simulink model "ObstacleControl"  (R2020a)
settings: Solver=ode3  StartTime=0.0  StopTime=10.0  RelTol=1e-3
PreLoadFcn:
  | % Lidar parameters
  | 
  | 
  | scanAngles = linspace(-pi/2,pi/2,360);
  | scanMaxRange = 3.5;
  | scanSensorOffset = [0,0];
model workspace (MAT data in the model file):
  destX = 2
  destY = 2
undefined symbols (not defined in the file or in its folder): Angular, Linear
libraries: robotlib x8, simulink x2, robotalgslib x2, robotcorelib x1
settings Model: Creator=Pierre  LastModifiedBy=pierre
settings OptimizationCC: EnhancedBackFolding=on  PassReuseOutputArgsAs=Individual arguments  ZeroExternalMemoryAtStartup=off  ZeroInternalMemoryAtStartup=off  MaxStackSize=64  OptimizeBlockOrder=speed  DifferentSizesBufferReuse=on  OptimizationCustomize=off  EfficientTunableParamExpr=on
settings DebuggingCC: ParameterTunabilityLossMsg=error
settings HardwareCC: ProdBitPerPointer=32  ProdBitPerSizeT=32  ProdBitPerPtrDiffT=32  ProdLargestAtomicFloat=None  ProdIntDivRoundTo=Undefined  ProdEndianess=Unspecified  ProdWordSize=32  ProdHWDeviceType=Generic->Unspecified (assume 32-bit Generic)
settings SFSimCC: MATLABDynamicMemAlloc=off
settings RTWCC: SystemTargetFile=ert.tlc  HardwareBoard=Robot Operating System (ROS)  TemplateMakefile=ert_default_tmf  Toolchain=Catkin  TargetLang=C++
settings CodeAppCC: ForceParamTrailComments=on  IgnoreCustomStorageClasses=off  OperatorAnnotations=on  SimulinkDataObjDesc=on  SFDataObjDesc=on  InsertBlockDesc=on
settings ERTTargetCC: SupportVariableSizeSignals=on

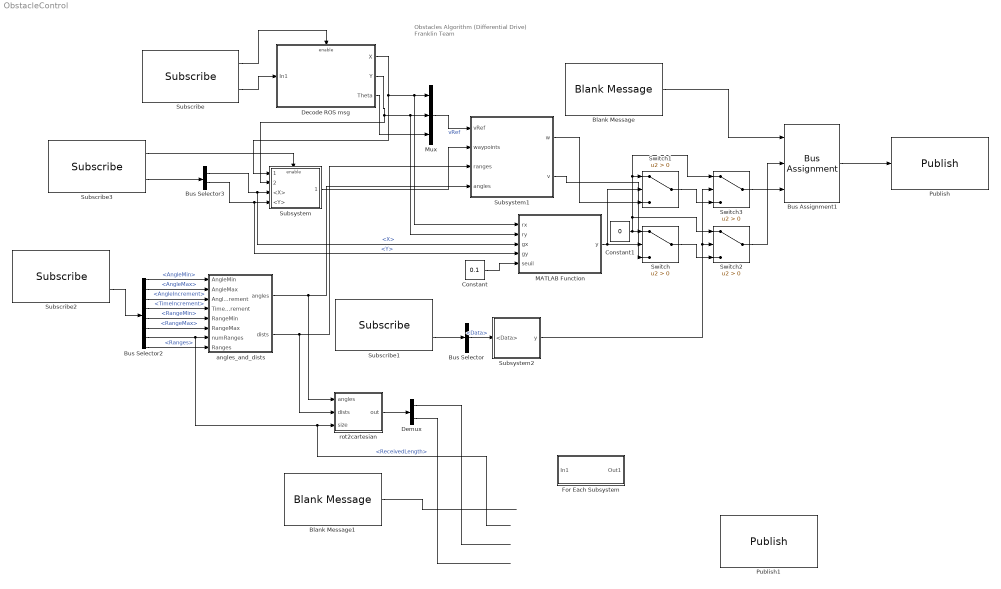
== system ObstacleControl ==
  note: Obstacles Algorithm
      | (Differential Drive)
      |
      | Franklin Team
  Blank Message : robotlib/Blank Message  messageClass=Message  entityType=geometry_msgs/Twist  messageType=geometry_msgs/Twist  SampleTime=inf
  Blank Message1 : robotlib/Blank Message  messageClass=Message  entityType=sensor_msgs/PointCloud  messageType=sensor_msgs/PointCloud  SampleTime=inf
  Bus Assignment1 : BusAssignment  AssignedSignals=Linear.X,Angular.Z
  Bus Selector : BusSelector  DialogController=Simulink.DDGSource_BusSelector  OutputSignals=Data
  Bus Selector2 : BusSelector  OutputSignals=AngleMin,AngleMax,AngleIncrement,TimeIncrement,RangeMin,RangeMax,Ranges_SL_Info.ReceivedLength,Ranges
  Bus Selector3 : BusSelector  OutputSignals=X,Y
  Constant : Constant  Value=0.1
  Constant1 : Constant  Value=0
  Decode ROS msg : Subsystem
  Demux : Demux  Outputs=2
  For Each Subsystem : Subsystem  TreatAsAtomicUnit=on
  MATLAB Function : MATLAB Function  TreatAsAtomicUnit=on
  Mux : Mux  Inputs=3
  Publish : robotlib/Publish  topicSource=Specify your own  topic=/cmd_vel  messageType=geometry_msgs/Twist  messageQueueLength=1
  Publish1 : robotlib/Publish  topicSource=Specify your own  topic=/modelScan  messageType=sensor_msgs/PointCloud  messageQueueLength=1
  Subscribe : robotlib/Subscribe  topicSource=Specify your own  topic=/odom  messageType=nav_msgs/Odometry  sampleTime=-1  messageQueueLength=1
  Subscribe1 : robotlib/Subscribe  topicSource=Specify your own  topic=/destination/stop  messageType=std_msgs/Bool  sampleTime=1  messageQueueLength=1
  Subscribe2 : robotlib/Subscribe  topicSource=Specify your own  topic=/scan  messageType=sensor_msgs/LaserScan  sampleTime=1  messageQueueLength=1
  Subscribe3 : robotlib/Subscribe  topicSource=Specify your own  topic=/destination  messageType=geometry_msgs/Pose2D  sampleTime=1  messageQueueLength=1
  Subsystem : Subsystem
  Subsystem1 : Subsystem
  Subsystem2 : Subsystem
  Switch{,1..3} (4 alike) : Switch  Criteria=u2 > Threshold
  angles_and_dists : MATLAB Function  TreatAsAtomicUnit=on
  rot2cartesian : MATLAB Function  TreatAsAtomicUnit=on
  wires:
  Blank Message/1 -> Bus Assignment1/1
  Bus Assignment1/1 -> Publish/1
  Subscribe3/2 -> Bus Selector3/1
  Subscribe3/1 -> Subsystem/Enable
  Subscribe/2 -> Decode ROS msg/1(In1)
  Subscribe/1 -> Decode ROS msg/Enable
  Decode ROS msg/1(X) -> Subsystem/1(<Xinit>), MATLAB Function/1(rx), Mux/1
  Decode ROS msg/2(Y) -> Subsystem/2(<Yinit>), MATLAB Function/2(ry), Mux/2
  Decode ROS msg/3(Theta) -> Mux/3
  Bus Selector3/1 -> MATLAB Function/3(gx), Subsystem/3(<X>)  "<X>"
  Bus Selector3/2 -> MATLAB Function/4(gy), Subsystem/4(<Y>)  "<Y>"
  Constant/1 -> MATLAB Function/5(seuil)
  MATLAB Function/1(y) -> Switch1/2, Switch/2
  Constant1/1 -> Switch2/1, Switch3/1, Switch1/1, Switch/1
  Switch/1 -> Switch2/3
  Switch2/1 -> Bus Assignment1/2
  Switch1/1 -> Switch3/3
  Switch3/1 -> Bus Assignment1/3
  Subscribe1/2 -> Bus Selector/1
  Subsystem2/1(y) -> Switch2/2, Switch3/2
  Bus Selector/1 -> Subsystem2/1(<Data>)  "<Data>"
  Subscribe2/2 -> Bus Selector2/1
  Mux/1 -> Subsystem1/1(vRef)  "vRef"
  Subsystem/1(waypoints) -> Subsystem1/2(waypoints)
  Subsystem1/1(w) -> Switch1/3
  Subsystem1/2(v) -> Switch/3
  Bus Selector2/6 -> angles_and_dists/6(RangeMax)  "<RangeMax>"
  Bus Selector2/2 -> angles_and_dists/2(AngleMax)  "<AngleMax>"
  Bus Selector2/3 -> angles_and_dists/3(AngleIncrement)  "<AngleIncrement>"
  Bus Selector2/5 -> angles_and_dists/5(RangeMin)  "<RangeMin>"
  Bus Selector2/7 -> rot2cartesian/3(size), angles_and_dists/7(numRanges)  "<ReceivedLength>"
  Bus Selector2/8 -> angles_and_dists/8(Ranges)  "<Ranges>"
  Bus Selector2/1 -> angles_and_dists/1(AngleMin)  "<AngleMin>"
  Bus Selector2/4 -> angles_and_dists/4(TimeIncrement)  "<TimeIncrement>"
  angles_and_dists/2(dists) -> rot2cartesian/2(dists), Subsystem1/3(ranges)
  angles_and_dists/1(angles) -> rot2cartesian/1(angles), Subsystem1/4(angles)
  Blank Message1/1 -> ?
  rot2cartesian/1(out) -> Demux/1
  Demux/1 -> ?
  Demux/2 -> ?
  ? -> Publish1/1

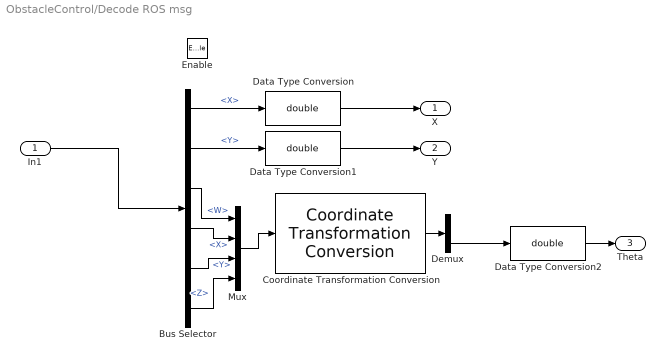
== system ObstacleControl/Decode ROS msg ==
  In1 : Inport
  Enable : EnablePort
  Bus Selector : BusSelector  DialogController=Simulink.DDGSource_BusSelector  OutputSignals=Pose.Pose.Position.X,Pose.Pose.Position.Y,Pose.Pose.Orientation.W,Pose.Pose.Orientation.X,Pose.Pose.Orientation.Y,Pose.Pose.Orientation.Z
  Coordinate Transformation Conversion : robotcorelib/Coordinate Transformation Conversion  InputRepresentation=Quaternion  InputEulerSequence=ZYX  ShowTrVecInputPort=on  OutputRepresentation=Euler Angles  OutputEulerSequence=XYZ  ShowTrVecOutputPort=on  SimulateUsing=Interpreted execution
      settings: SourceProductBaseCode=NV,RO,RR
  Data Type Conversion : DataTypeConversion  OutDataTypeStr=double
  Data Type Conversion1 : DataTypeConversion  OutDataTypeStr=double
  Data Type Conversion2 : DataTypeConversion  OutDataTypeStr=double
  Demux : Demux  Outputs=3
  Mux : Mux
  X : Outport  VectorParamsAs1DForOutWhenUnconnected=off
  Y : Outport  Port=2  VectorParamsAs1DForOutWhenUnconnected=off
  Theta : Outport  Port=3  VectorParamsAs1DForOutWhenUnconnected=off
  wires:
  In1/1 -> Bus Selector/1
  Bus Selector/2 -> Data Type Conversion1/1  "<Y>"
  Bus Selector/1 -> Data Type Conversion/1  "<X>"
  Data Type Conversion/1 -> X/1
  Data Type Conversion1/1 -> Y/1
  Data Type Conversion2/1 -> Theta/1
  Bus Selector/3 -> Mux/1  "<W>"
  Bus Selector/4 -> Mux/2  "<X>"
  Bus Selector/5 -> Mux/3  "<Y>"
  Bus Selector/6 -> Mux/4  "<Z>"
  Mux/1 -> Coordinate Transformation Conversion/1
  Coordinate Transformation Conversion/1 -> Demux/1
  Demux/3 -> Data Type Conversion2/1

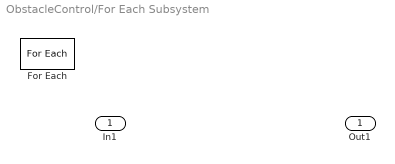
== system ObstacleControl/For Each Subsystem ==
  In1 : Inport  Partition=on  PartitionDimension=1  PartitionWidth=1  PartitionOffset=0
  For Each : ForEach  DisableCoverage=on
  Out1 : Outport  ConcatenationDimension=1

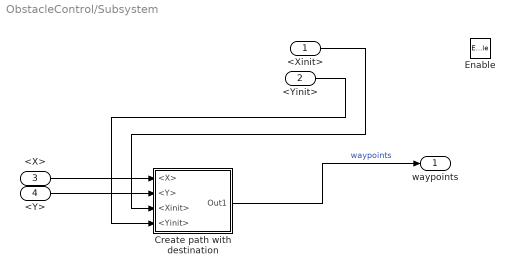
== system ObstacleControl/Subsystem ==
  <Xinit> : Inport
  <Yinit> : Inport  Port=2
  <X> : Inport  Port=3
  <Y> : Inport  Port=4
  Enable : EnablePort
  Create path with destination : Subsystem
  waypoints : Outport
  wires:
  <Yinit>/1 -> Create path with destination/4(<Yinit>)
  <X>/1 -> Create path with destination/1(<X>)
  <Y>/1 -> Create path with destination/2(<Y>)
  Create path with destination/1(Out1) -> waypoints/1  "waypoints"
  <Xinit>/1 -> Create path with destination/3(<Xinit>)

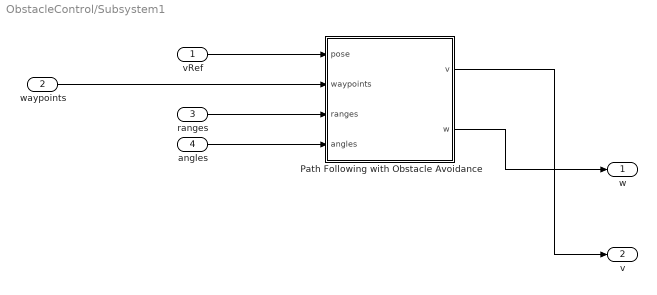
== system ObstacleControl/Subsystem1 ==
  vRef : Inport
  waypoints : Inport  Port=2
  ranges : Inport  Port=3
  angles : Inport  Port=4
  Path Following with Obstacle Avoidance : Subsystem
  w : Outport
  v : Outport  Port=2
  wires:
  vRef/1 -> Path Following with Obstacle Avoidance/1(pose)
  Path Following with Obstacle Avoidance/2(w) -> w/1
  waypoints/1 -> Path Following with Obstacle Avoidance/2(waypoints)
  Path Following with Obstacle Avoidance/1(v) -> v/1
  ranges/1 -> Path Following with Obstacle Avoidance/3(ranges)
  angles/1 -> Path Following with Obstacle Avoidance/4(angles)

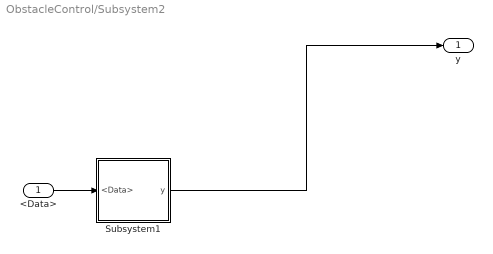
== system ObstacleControl/Subsystem2 ==
  <Data> : Inport
  Subsystem1 : Subsystem
  y : Outport
  wires:
  Subsystem1/1(y) -> y/1
  <Data>/1 -> Subsystem1/1(<Data>)

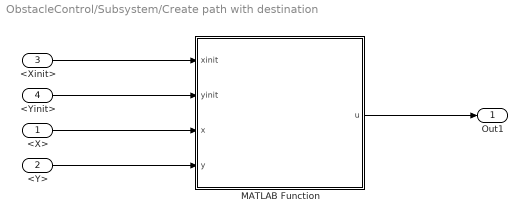
== system ObstacleControl/Subsystem/Create path with destination ==
  <X> : Inport
  <Y> : Inport  Port=2
  <Xinit> : Inport  Port=3
  <Yinit> : Inport  Port=4
  MATLAB Function : MATLAB Function  TreatAsAtomicUnit=on
  Out1 : Outport
  wires:
  <Y>/1 -> MATLAB Function/4(y)
  <X>/1 -> MATLAB Function/3(x)
  MATLAB Function/1(u) -> Out1/1
  <Xinit>/1 -> MATLAB Function/1(xinit)
  <Yinit>/1 -> MATLAB Function/2(yinit)

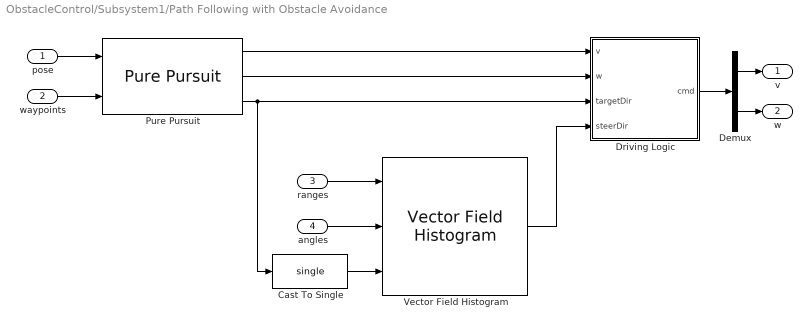
== system ObstacleControl/Subsystem1/Path Following with Obstacle Avoidance ==
  pose : Inport
  waypoints : Inport  Port=2
  ranges : Inport  Port=3
  angles : Inport  Port=4
  Cast To Single : DataTypeConversion  OutDataTypeStr=single
  Demux : Demux  Outputs=2
  Driving Logic : Subsystem
  Pure Pursuit : robotalgslib/Pure Pursuit  DesiredLinearVelocity=0.1  MaxAngularVelocity=1.5  LookaheadDistance=0.2  TargetDirPort=on  SimulateUsing=Interpreted execution
      settings: SourceProductBaseCode=RO
  Vector Field Histogram : robotalgslib/Vector Field Histogram  NumAngularSectors=36  DistanceLimits=[ 0.05, 3 ]  HistogramThresholds=[ 5, 10 ]  RobotRadius=0.1  SafetyDistance=0.2  MinTurningRadius=0.25  SimulateUsing=Interpreted execution  TargetDirectionWeight=5  CurrentDirectionWeight=2  PreviousDirectionWeight=2
      settings: SourceProductBaseCode=RO
  v : Outport  VectorParamsAs1DForOutWhenUnconnected=off
  w : Outport  Port=2  VectorParamsAs1DForOutWhenUnconnected=off
  wires:
  pose/1 -> Pure Pursuit/1
  Pure Pursuit/3 -> Driving Logic/3(targetDir), Cast To Single/1
  Pure Pursuit/1 -> Driving Logic/1(v)
  angles/1 -> Vector Field Histogram/2
  Vector Field Histogram/1 -> Driving Logic/4(steerDir)
  ranges/1 -> Vector Field Histogram/1
  waypoints/1 -> Pure Pursuit/2
  Pure Pursuit/2 -> Driving Logic/2(w)
  Demux/1 -> v/1
  Demux/2 -> w/1
  Driving Logic/1(cmd) -> Demux/1
  Cast To Single/1 -> Vector Field Histogram/3

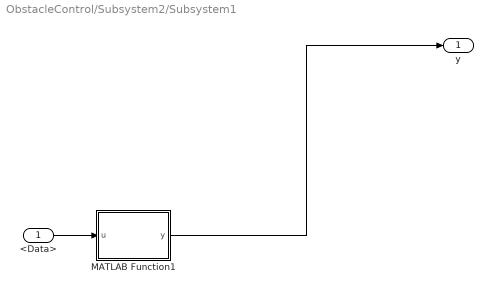
== system ObstacleControl/Subsystem2/Subsystem1 ==
  <Data> : Inport
  MATLAB Function1 : MATLAB Function  TreatAsAtomicUnit=on
  y : Outport
  wires:
  <Data>/1 -> MATLAB Function1/1(u)
  MATLAB Function1/1(y) -> y/1

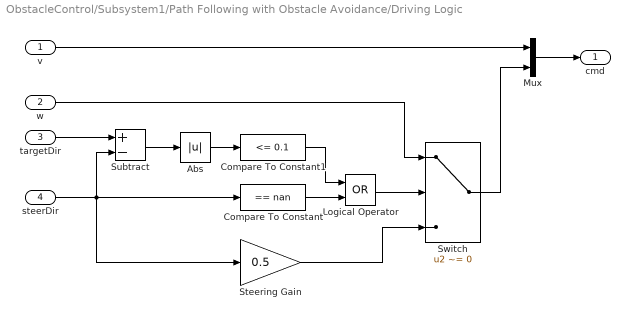
== system ObstacleControl/Subsystem1/Path Following with Obstacle Avoidance/Driving Logic ==
  v : Inport
  w : Inport  Port=2
  targetDir : Inport  Port=3
  steerDir : Inport  Port=4
  Abs : Abs
  Compare To Constant : simulink/Logic and Bit Operations/Compare To Constant  relop===  const=nan  OutDataTypeStr=boolean
  Compare To Constant1 : simulink/Logic and Bit Operations/Compare To Constant  relop=<=  const=0.1  OutDataTypeStr=boolean
  Logical Operator : Logic  Operator=OR  AllPortsSameDT=off  OutDataTypeStr=boolean
  Mux : Mux  Inputs=2
  Steering Gain : Gain  Gain=0.5
  Subtract : Sum  Inputs=+-
  Switch : Switch  Criteria=u2 ~= 0
  cmd : Outport  VectorParamsAs1DForOutWhenUnconnected=off
  wires:
  v/1 -> Mux/1
  steerDir/1 -> Steering Gain/1, Subtract/2, Compare To Constant/1
  Compare To Constant/1 -> Logical Operator/2
  targetDir/1 -> Subtract/1
  Subtract/1 -> Abs/1
  Abs/1 -> Compare To Constant1/1
  Compare To Constant1/1 -> Logical Operator/1
  Mux/1 -> cmd/1
  Logical Operator/1 -> Switch/2
  w/1 -> Switch/1
  Switch/1 -> Mux/2
  Steering Gain/1 -> Switch/3

== matlab function ObstacleControl/MATLAB Function ==
  data: rx input; y output; ry input; gx input; gy input; seuil input
function y = detectGoal(rx, ry, gx, gy, seuil)
posDiff = [gx-rx;gy-ry];
dist = sqrt(posDiff(1)^2 + posDiff(2)^2);

if dist <= seuil
    y = 1;
else
    y = 0;
end

== matlab function ObstacleControl/Subsystem/Create path with destination/MATLAB Function ==
  data: xinit input; yinit input; x input; y input; u output
function u = newDest(xinit, yinit, x, y)
u = [xinit,yinit; x,y];

== matlab function ObstacleControl/Subsystem2/Subsystem1/MATLAB Function1 ==
  data: u input; y output
function y = boolToInt(u)
if u == 1
    y = 1;
else
    y = 0;
end

== matlab function ObstacleControl/rot2cartesian ==
  data: angles input; dists input; size input; out output
function out = fcn(angles,dists,size)
%#codegen
% x values align with "forward" points
xs = dists.*cos(angles);
% y values align with left (positive) points
ys = dists.*sin(angles);
points = [xs,ys];
out = points;

== matlab function ObstacleControl/angles_and_dists ==
  data: AngleMin input size=1 [-2*pi..2*pi]; angles output size=[180 1]; dists output size=[180 1]; AngleMax input [-2*pi..2*pi]; AngleIncrement input [0..2*pi]; TimeIncrement input; RangeMin input; RangeMax input; numRanges input [1..360]; Ranges input
function [angles,dists] = fcn(AngleMin, AngleMax, AngleIncrement, ...
                TimeIncrement, RangeMin, RangeMax, numRanges, Ranges )
%#codegen
% this function transforms the laser scan into cartesian coordinates, so
% that you can use other tools to group them together, make an image, etc.
if numRanges > 0 
angleMin = double(AngleMin);
angleMax = double(AngleMax);
angleIncrement = double(AngleIncrement);
% assert(angleMax > angleMin);
% assert((angleMax-angleMin)/angleIncrement > 1);
% 
% angleMin = -pi/2;
% angleMax = pi/2;
% angleIncrement = pi/179;
timeIncrement = TimeIncrement;
rangeMin = RangeMin;
rangeMax = RangeMax;
ranges = Ranges;
ranges(ranges>RangeMax) = NaN;
ranges(ranges<RangeMin) = NaN;
%rangesLength = scan.Ranges_SL_Info.ReceivedLength;
%intensities = scan.Intensities;
%coder.varsize('angles',[180 1]);

angles=double(zeros(numRanges,1));
for ii=1:numRanges
    angles(ii) = double(angleMin) + double(ii-1)*(angleIncrement);
end
% angles = [angleMin:angleIncrement:angleMax]';
dists = ranges;
else
    angles=double(0);
    dists=single(0);
end
